simulink model "CR"  (R2024a)
settings: Solver=VariableStepAuto  StartTime=0.0  StopTime=inf  FixedStep=0.01  RelTol=1e-3
undefined symbols (not defined in the file or in its folder): QAM
libraries: simulink x4, commrandsrc3 x2, commdigbbndam3 x2, dspxfrm3 x1, commchan3 x1, commsink2 x1, sdrrlib x1, rtlsdr_book_library x1, rfmathmodels2 x1, commfilt2 x1
settings Model: Creator=aukustiharris  LastModifiedBy=aukustiharris
settings SolverCC: AlgebraicLoopSolver=TrustRegion  AutoInsertRateTranBlk=on
settings DataIOCC: LimitDataPoints=on  SaveOutput=off  SaveTime=off
settings OptimizationCC: BooleanDataType=off  DefaultParameterBehavior=Inlined  LocalBlockOutputs=off  LifeSpan=inf
settings DebuggingCC: AlgebraicLoopMsg=error  SingleTaskRateTransMsg=error  UnconnectedInputMsg=warning  UnconnectedOutputMsg=warning  UnconnectedLineMsg=warning  AllowSymbolicDim=off  SFUnexpectedBacktrackingDiag=warning  SFNoUnconditionalDefaultTransitionDiag=warning  SFExecutionAtInitializationDiag=none  ArithmeticOperatorsInVariantConditions=warning
settings ModelReferenceCC: EnableRefExpFcnMdlSchedulingChecks=on
settings SFSimCC: SimUseLocalCustomCode=off  CustomCodeUndefinedFunction=UseInterfaceOnly
settings RTWCC: RTWUseLocalCustomCode=off  GPUComputeCapability=3.5
settings CodeAppCC: StateflowObjectComments=on
settings GRTTargetCC: TargetLangStandard=C89/C90 (ANSI)
settings ConfigComp: CovMetricSettings=dw  CovSaveCumulativeToWorkspaceVar=on  CovSaveSingleToWorkspaceVar=on  CovExternalEMLEnable=off  CovSFcnEnable=off

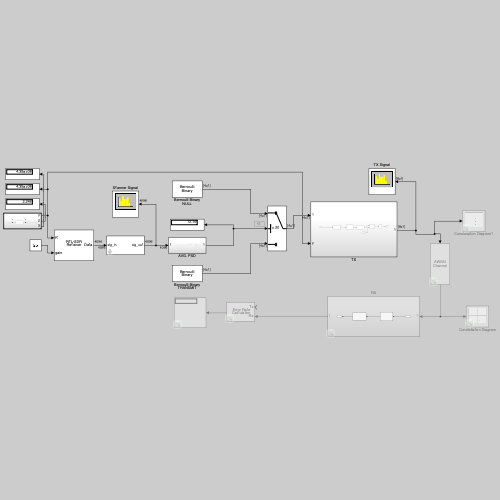
[thumbnail: Simulink's stored preview of the top-level diagram]
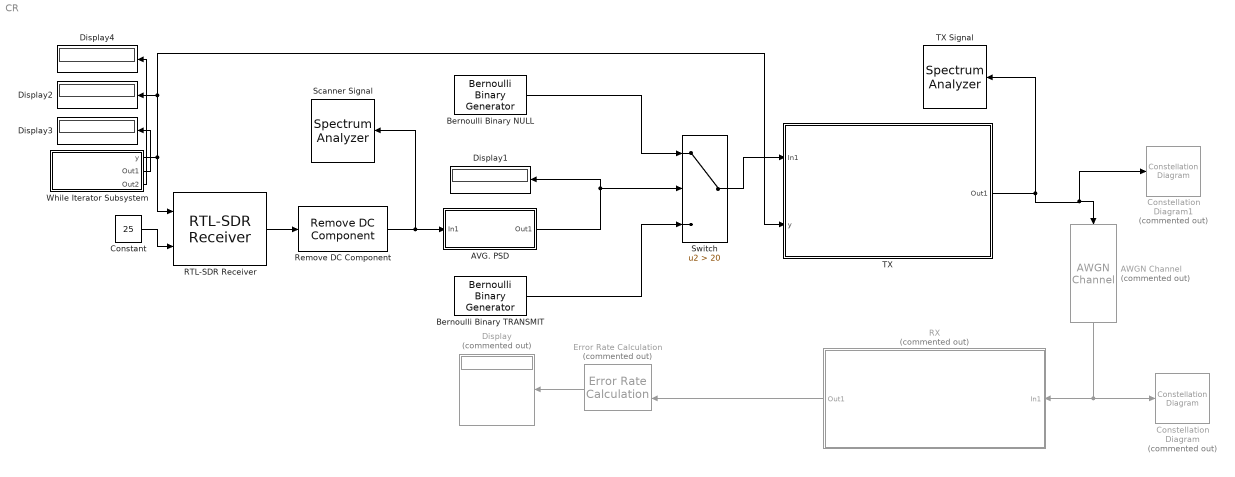
== system CR ==
  AVG. PSD : Subsystem
  AWGN Channel : commchan3/AWGN Channel  Commented=on  LegacyMode=off  NoiseMethod="Signal to noise ratio  (SNR)"  noiseMode="Signal to noise ratio  (SNR)"  EbNo=10  EsNo=10  SNR=10  BitsPerSymbol=1  SignalPower=1  SamplesPerSymbol=1  SymbolPeriod=1  VarianceSource=Parameter  Variance=1  RandomStream=Global stream  Seed=67  SimulateUsing=Code generation
  Bernoulli Binary NULL : commrandsrc3/Bernoulli Binary Generator  ProbabilityOfZero=1  SeedSource=Parameter  Seed=61  SampleTime=1/1e6  SamplesPerFrame=log2(16)  OutputDataType=single  SimulateUsing=Interpreted execution
  Bernoulli Binary TRANSMIT : commrandsrc3/Bernoulli Binary Generator  ProbabilityOfZero=0.5  SeedSource=Parameter  Seed=61  SampleTime=1/1e6  SamplesPerFrame=log2(16)  OutputDataType=single  SimulateUsing=Interpreted execution
  Constant : Constant  Value=25
  Constellation Diagram : ConstellationDiagram  Commented=on  WindowPosition=[-1876.000000,515.000000,571.000000,503.000000,]  ScopeFrameLocation=window  SymbolsToDisplaySource=Property  SymbolsToDisplay=200  ReferenceConstellation=16-QAM  XLimits=[-1.46,1.46]  YLimits=[-1.53,1.53]
  Constellation Diagram1 : ConstellationDiagram  Commented=on  WindowPosition=[-1883.000000,17.000000,570.000000,497.000000,]  ScopeFrameLocation=window  SymbolsToDisplaySource=Property  SymbolsToDisplay=200  ReferenceConstellation=16-QAM  XLimits=[-3.36,5.24]  YLimits=[-2.41,1.93]  ShowReferenceConstellation=off
  Display : Display  Commented=on
  Display{1..4} (4 alike) : Display
  Error Rate Calculation : commsink2/Error Rate Calculation  Commented=on  N=0  st_delay=0  cp_mode=Entire frame  subframe=[]  PMode=Port  WsName=ErrorVec  RsMode2=off  stop=off  numErr=100  maxBits=1e6
  RTL-SDR Receiver : sdrrlib/RTL-SDR Receiver  IPAddress=0  CenterFrequencySource=Input port  CenterFrequency=435e6  GainSource=Input port  Gain=0  ADCRate=2.4e6  FrequencyCorrection=0  LostSamplesOutputPort=off  LatencyOutputPort=off  OutputDataType=single  FrameLength=4096  EnableBurstMode=off  NumFramesInBurst=20  sobjType=sdrr.internal.SDRRTLReceiverSL  dataUDPPort=-1  ctrlUDPPort=-1  subDeviceList=nosubdev  sdrBlockType=SDRBlockTypeSLT.SDRRxBlock  requester=UNUSED_BY_SFCN  sdrExecutionMode=SDRExecutionModeSLT.ExecModeHW  BypassUserLogic=off  DecimatorSelect=DDC decimator  SourceSelect=RF data  SineAmplitude=16000  EnableInternalClock=off  BypassIQBalance=off  IFBandwidth=40e6  ADCRateSource=Dialog  IntermediateFrequency=0  DecimationFactorSource=Dialog  DecimationFactor=512  RFFrequencyIsTunable=logical(1)  SampleTime=(4096)/(2.4e6)  IFBandwidthSource=Dialog  SineFrequency=30000  BypassDCBlockingFilter=off  IntermediateFrequencySource=Dialog  IQBalanceCoefficients=64  SkipAllHardwareResetAndInitialization=off  EnableIQCalibrationTable=on  CacheIQCalibrationTable=off  EnableOffsetTuning=off  EnableRTLAGC=off  EnableTestMode=off  EnableTunerAGC=off  FrequencyCorrectionSource=Dialog  NumMLBuffers=128  NumUSBBuffers=16  RTLCrystalFrequency=28800000  TunerCrystalFrequency=28800000
  RX : Subsystem  Commented=on
  Remove DC Component : rtlsdr_book_library/Additional Tools/Remove DC Component
      settings: SourceProductName=RTL-SDR Book Library
  Scanner Signal : SpectrumAnalyzer  Tag=simrfV2util1/Spectrum Analyzer  WindowPosition=[-1912.000000,8.000000,949.000000,1011.000000,]  ScopeFrameLocation=window  Method=Welch  AxesScaling=Manual  FrequencyResolutionMethod=Window length  WindowLength=4096  Span=2800000  StartFrequency=-1400000  StopFrequency=1400000  AveragingMethod=Exponential  YLimits=[-40 10]  ColorLimits=[-37.215302,-12.67160075]  AllowFFTLengthLessThanSamplesPerUpdate=on
  Switch : Switch  Criteria=u2 > Threshold  Threshold=20  OutDataTypeStr=single  SaturateOnIntegerOverflow=off
      settings: LockScale=on
  TX : Subsystem
  TX Signal : SpectrumAnalyzer  Tag=simrfV2util1/Spectrum Analyzer  WindowPosition=[-954.000000,9.000000,948.000000,1011.000000,]  ScopeFrameLocation=window  Method=Welch  AxesScaling=Manual  FrequencyResolutionMethod=Window length  WindowLength=4096  Span=2800000  StartFrequency=-1400000  StopFrequency=1400000  AveragingMethod=Exponential  YLimits=[-15,10]  ColorLimits=[-37.215302,-12.67160075]  AllowFFTLengthLessThanSamplesPerUpdate=on
  While Iterator Subsystem : Subsystem  TreatAsAtomicUnit=on
  wires:
  TX/1(Out1) -> AWGN Channel/1, Constellation Diagram1/1, TX Signal/1
  RX/1(Out1) -> Error Rate Calculation/2
  Error Rate Calculation/1 -> Display/1
  AVG. PSD/1(Out1) -> Display1/1, Switch/2
  RTL-SDR Receiver/1 -> Remove DC Component/1
  Remove DC Component/1 -> Scanner Signal/1, AVG. PSD/1(In1)
  Bernoulli Binary TRANSMIT/1 -> Switch/3
  Bernoulli Binary NULL/1 -> Switch/1
  Switch/1 -> TX/1(In1)
  Constant/1 -> RTL-SDR Receiver/2
  AWGN Channel/1 -> Constellation Diagram/1, RX/1(In1)
  While Iterator Subsystem/1(y) -> RTL-SDR Receiver/1, TX/2(y), Display2/1
  While Iterator Subsystem/2(Out1) -> Display3/1
  While Iterator Subsystem/3(Out2) -> Display4/1

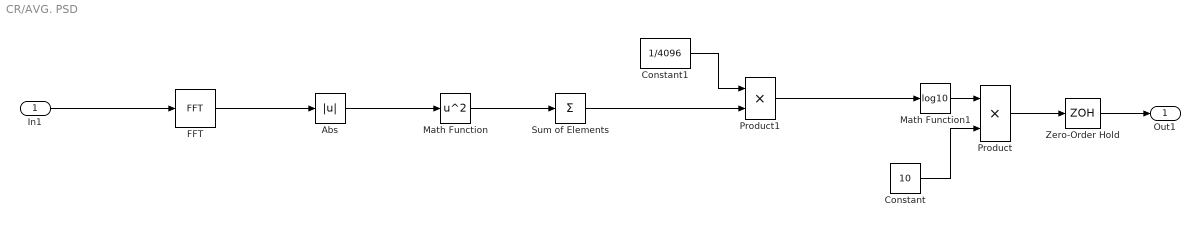
== system CR/AVG. PSD ==
  In1 : Inport
  Abs : Abs  OutDataTypeStr=single  SaturateOnIntegerOverflow=off
  Constant : Constant  Value=10
  Constant1 : Constant  Value=1/4096
  FFT : dspxfrm3/FFT  FFTImplementation=Auto  CompMethod=Table lookup  TableOpt=NEW  TableOptActive=Speed  BitRevOrder=off  Normalize=off  InheritFFTLength=on  FFTLength=64  WrapInput=on  roundingMode=Ceiling  overflowMode=off  firstCoeffDataTypeStr=Inherit: Same word length as input  firstCoeffLastDataTypeStr=Inherit: Same word length as input  outputMin=[]  outputMax=[]
  Math Function : Math  Operator=square  OutDataTypeStr=single
  Math Function1 : Math  Operator=log10
  Product : Product
  Product1 : Product
  Sum of Elements : Sum  Inputs=+  AccumDataTypeStr=single
  Zero-Order Hold : ZeroOrderHold  SampleTime=0.001
  Out1 : Outport
  wires:
  FFT/1 -> Abs/1
  Abs/1 -> Math Function/1
  In1/1 -> FFT/1
  Math Function1/1 -> Product/1
  Constant/1 -> Product/2
  Math Function/1 -> Sum of Elements/1
  Sum of Elements/1 -> Product1/2
  Product1/1 -> Math Function1/1
  Constant1/1 -> Product1/1
  Zero-Order Hold/1 -> Out1/1
  Product/1 -> Zero-Order Hold/1

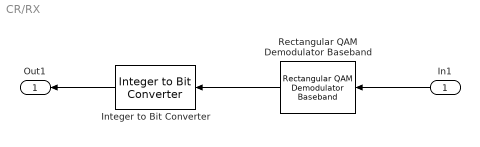
== system CR/RX ==
  In1 : Inport
  Integer to Bit Converter : simulink/Logic and Bit Operations/Integer to Bit Converter  nbits=4  signedInputValues=Unsigned  bitOrder=MSB first  outDtype=Inherit via internal rule
      settings: LibrarySourceBlock=|
      | commutil2/Integer to Bit
      | Converter
  Rectangular QAM Demodulator Baseband : commdigbbndam3/Rectangular QAM Demodulator Baseband  M=16  OutType=Integer  DecType=Hard decision  VarSource=Dialog  Variance=1  Dec=Gray  Mapping=[0:15]  PowType=Average Power  MinDist=2  AvgPow=1  PeakPow=1  Ph=0  outDtype1=Inherit via internal rule  outDtype2=single  derotateFactorWordLen=16  derotateFactorDataTypeStr=Inherit: Same word length as input  derotateFactorLastDataTypeStr=Inherit: Same word length as input  denormFactorWordLen=16  denormFactorDataTypeStr=Inherit: Same word length as input  denormFactorLastDataTypeStr=Inherit: Same word length as input  prodOutWordLen=32  prodOutOverflowMode=Wrap  prodOutRoundingMode=Floor  prodOutOvFlMode=off  prodOutOvFlModeLastStrValue=off  sumWordLen=32
  Out1 : Outport
  wires:
  In1/1 -> Rectangular QAM Demodulator Baseband/1
  Rectangular QAM Demodulator Baseband/1 -> Integer to Bit Converter/1
  Integer to Bit Converter/1 -> Out1/1

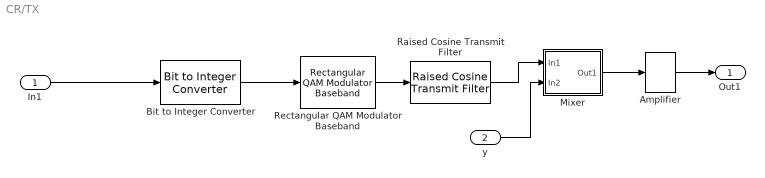
== system CR/TX ==
  In1 : Inport
  y : Inport  Port=2
  Amplifier : rfmathmodels2/Amplifier  Model=Cubic polynomial  LinearGainDB=0  TOI_Type=IIP3  IIP3=Inf  OIP3=Inf  IP1dB=Inf  OP1dB=Inf  IPsat=Inf  OPsat=Inf  Table="[-25,    5,   -1;  -10,   20,   -2;  0,   27,    5;  5,   28,   12]"  MagnitudeGainDB=0  Vsat=1  MagnitudeSmooth=2  PhaseGainRadian=-.45  PhaseSaturation=.88  PhaseSmooth=3.43  InputScaleDB=0  AmAmParameters=[ 2.1587, 1.1517 ]  AmPmParameters=[ 4.0033, 9.1040 ]  OutputScaleDB=0  SimulateUsing=Interpreted execution  IncludeNoise=off  NoiseType=Noise temperature  NoiseTemperature=290  NoiseFigure=10 * log10( 2 )  NoiseFactor=2  SeedSource=Auto  Seed=67987
  Bit to Integer Converter : simulink/Logic and Bit Operations/Bit to Integer Converter  nbits=4  bitOrder=MSB first  signedOutputValues=Unsigned  outDtype=single  outDtypeSigned=Inherit via internal rule
  Mixer : Subsystem
  Raised Cosine Transmit Filter : commfilt2/Raised Cosine Transmit Filter  filtType=Square root  R=0.2  filtSpan=10  N=8  filterGain=1  InputProcessing=Columns as channels (frame based)  RateOptions=Enforce single-rate processing  framing=Mute  checkCoeff=off  variableName=rcTxFilt  checkGain=Normalized  sampMode=Mute  saveAsFlag=0  currentFiltSpan=10  D=(10)/2  launchFVT=on  roundingMode=Floor  overflowMode=off  coeffDataTypeStr=Inherit: Same word length as input  coeffMin=[]  coeffMax=[]  coeffLastDataTypeStr=Inherit: Same word length as input  outputDataTypeStr=Inherit: Same as accumulator  outputMin=[]  outputMax=[]  outputLastDataTypeStr=Inherit: Same as accumulator
  Rectangular QAM Modulator Baseband : commdigbbndam3/Rectangular QAM Modulator Baseband  M=16  InType=Integer  Enc=Gray  Mapping=[0:15]  PowType=Average Power  MinDist=2  AvgPow=1  PeakPow=1  Ph=0  outDtype=double  outWordLen=16  outUDDataType=sfix(16)  outFracLenMode=Best precision  outFracLen=15  outDataTypeStr=double  outLastDataTypeStr=double
  Out1 : Outport
  wires:
  Bit to Integer Converter/1 -> Rectangular QAM Modulator Baseband/1
  In1/1 -> Bit to Integer Converter/1
  Rectangular QAM Modulator Baseband/1 -> Raised Cosine Transmit Filter/1
  y/1 -> Mixer/2(In2)
  Raised Cosine Transmit Filter/1 -> Mixer/1(In1)
  Amplifier/1 -> Out1/1
  Mixer/1(Out1) -> Amplifier/1

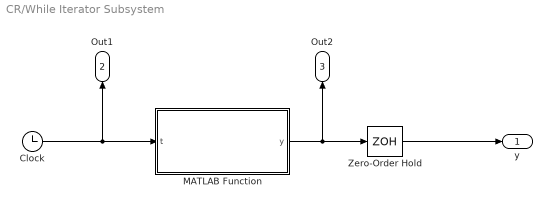
== system CR/While Iterator Subsystem ==
  Clock : Clock
  MATLAB Function : MATLAB Function  TreatAsAtomicUnit=on
  Zero-Order Hold : ZeroOrderHold  SampleTime=-1
  y : Outport
  Out1 : Outport  Port=2
  Out2 : Outport  Port=3
  wires:
  Clock/1 -> Out1/1, MATLAB Function/1(t)
  MATLAB Function/1(y) -> Out2/1, Zero-Order Hold/1
  Zero-Order Hold/1 -> y/1

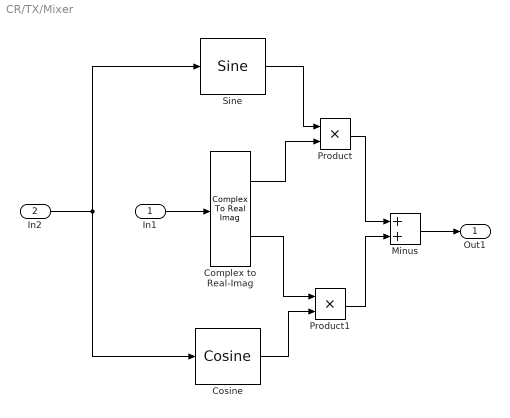
== system CR/TX/Mixer ==
  In1 : Inport
  In2 : Inport  Port=2
  Complex to Real-Imag : ComplexToRealImag
  Cosine : simulink/Lookup Tables/Cosine  Formula=sin(2*pi*u)  NumDataPoints=(2^5)+1  OutputWordLength=16  InternalRulePriority=Speed
  Minus : Sum
  Product : Product
  Product1 : Product
  Sine : simulink/Lookup Tables/Sine  Formula=cos(2*pi*u)  NumDataPoints=(2^5)+1  OutputWordLength=16  InternalRulePriority=Speed
  Out1 : Outport
  wires:
  In1/1 -> Complex to Real-Imag/1
  In2/1 -> Cosine/1, Sine/1
  Complex to Real-Imag/1 -> Product/2
  Sine/1 -> Product/1
  Complex to Real-Imag/2 -> Product1/1
  Cosine/1 -> Product1/2
  Product/1 -> Minus/1
  Product1/1 -> Minus/2
  Minus/1 -> Out1/1

== matlab function CR/While Iterator Subsystem/MATLAB Function ==
  data: y output; t input
function y = MATLAB_Function(t)
    % Array of center frequencies
    %centerFreq = [939515400, 941515400, 943515400, 945515400, 947515400];
    %centerFreq = 433000000:2e6:1700000000;
    %centerFreq = 795000000;
    centerFreq = 435000000; 
    % Define a persistent variable to hold the current index
    persistent freqIndex;
    persistent lastUpdate;
    
    % Initialize persistent variables on the first run
    if isempty(freqIndex)
        freqIndex = 1; % Start with the first frequency
    end
    if isempty(lastUpdate)
        lastUpdate = 0; % Last update time
    end
    
    % Define the update interval in seconds
    updateInterval = 0.1; 
    
    % Check if the update interval has passed
    if t - lastUpdate >= updateInterval
        % Update the last update time
        lastUpdate = t;
        
        % Increment the frequency index
        freqIndex = freqIndex + 1;
        
        % Wrap around if the index exceeds the number of frequencies
        if freqIndex > length(centerFreq)
            freqIndex = 1; % Loop back to the first frequency
        end
    end
    
    % Output the current frequency
    y = centerFreq(freqIndex);
end
